simulink model "throttleMask"  (R2022b)
settings: Solver=ode45  StartTime=0.0  StopTime=20  RelTol=1e-3  EnableMultiTasking=on
PreLoadFcn:
  | % Throttle body parameters
  | etc_plant_data;
  | 
  | % Input data
  | load throttle_input;
settings Model: Creator=jrivitus  LastModifiedBy=bensweet
settings SolverCC: AlgebraicLoopSolver=TrustRegion
settings DataIOCC: ExternalInput=[t, duty, direction]  LimitDataPoints=on  LoadExternalInput=on  SaveFormat=Array  ReturnWorkspaceOutputs=off
settings OptimizationCC: ExpressionDepthLimit=2147483647  LifeSpan=inf
settings DebuggingCC: UnconnectedInputMsg=warning  UnconnectedOutputMsg=warning  UnconnectedLineMsg=warning  PregeneratedLibrarySubsystemCodeDiagnostic=none  SFMachineParentedDataDiag=warning
settings HardwareCC: ProdBitPerPointer=32  ProdBitPerSizeT=32  ProdBitPerPtrDiffT=32  ProdLargestAtomicFloat=None  ProdIntDivRoundTo=Undefined  ProdEndianess=Unspecified  ProdWordSize=32  ProdHWDeviceType=32-bit Generic
settings ModelReferenceCC: EnableRefExpFcnMdlSchedulingChecks=on  PropagateSignalLabelsOutOfModel=off
settings SFSimCC: SimUseLocalCustomCode=off
settings RTWCC: RTWUseLocalCustomCode=off  DLArmComputeVersion=19.05
settings CodeAppCC: StateflowObjectComments=on
settings GRTTargetCC: TargetLangStandard=C89/C90 (ANSI)  CombineOutputUpdateFcns=off  GRTInterface=on
settings ConfigComp: CovMetricSettings=dw  CovSaveCumulativeToWorkspaceVar=on  CovSaveSingleToWorkspaceVar=on  CovExternalEMLEnable=off  CovSFcnEnable=off

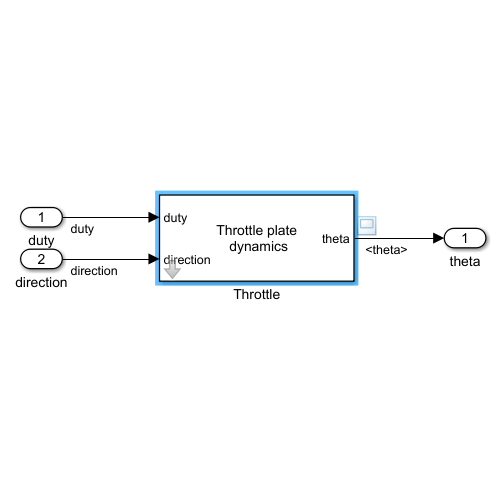
[thumbnail: Simulink's stored preview of the top-level diagram]
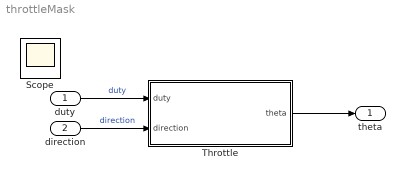
== system throttleMask ==
  duty : Inport
  direction : Inport  Port=2
  Throttle : Subsystem  mask(Throttle plate dynamics){J=2.45e-4, Km=3, Kd=0.03, Ks=0.2, theta_eq=pi/6}
      mask prompts: J "Inertia (J):"; Km "Motor torque constant (Km):"; Kd "Damping constant (Kd):"; Ks "Spring constant (Ks):"; theta_eq "Equilibrium angle (theta_eq):"
      mask help: Implements the dynamics for the throttle plate.
      mask Display: fprintf("Throttle plate\n dynamics")
  theta : Outport  VectorParamsAs1DForOutWhenUnconnected=off
  Scope : Scope
  wires:
  duty/1 -> Throttle/1(duty)  "duty"
  direction/1 -> Throttle/2(direction)  "direction"
  Throttle/1(theta) -> theta/1

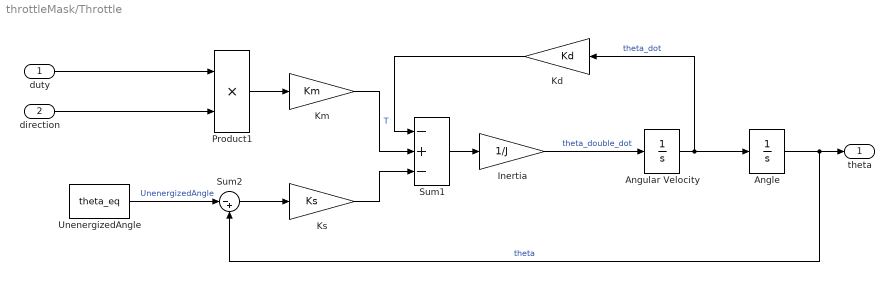
== system throttleMask/Throttle ==
  duty : Inport
  direction : Inport  Port=2
  Angle : Integrator  InitialCondition=pi/6  LimitOutput=on  UpperSaturationLimit=pi/2  LowerSaturationLimit=0
      settings: AttributesFormatString=Initial condition: %<InitialCondition>\n%<LowerSaturationLimit> <= theta <= %<UpperSaturationLimit>
  Angular Velocity : Integrator
      settings: AttributesFormatString=Initial condition: %<InitialCondition>
  Inertia : Gain  Gain=1/J  SaturateOnIntegerOverflow=on  OutDataTypeStr=Inherit: Same as input  ParamDataTypeStr=Inherit: Same as input
  Kd : Gain  Gain=Kd  SaturateOnIntegerOverflow=on  OutDataTypeStr=Inherit: Same as input  ParamDataTypeStr=Inherit: Same as input
  Km : Gain  Gain=Km  SaturateOnIntegerOverflow=on  OutDataTypeStr=Inherit: Same as input  ParamDataTypeStr=Inherit: Same as input
  Ks : Gain  Gain=Ks  SaturateOnIntegerOverflow=on  OutDataTypeStr=Inherit: Same as input  ParamDataTypeStr=Inherit: Same as input
  Product1 : Product  SaturateOnIntegerOverflow=on  OutDataTypeStr=Inherit: Same as first input
  Sum1 : Sum  Inputs=-+-  SaturateOnIntegerOverflow=on
  Sum2 : Sum  Inputs=|-+  SaturateOnIntegerOverflow=on
  UnenergizedAngle : Constant  Value=theta_eq
  theta : Outport  VectorParamsAs1DForOutWhenUnconnected=off
  wires:
  Product1/1 -> Km/1
  UnenergizedAngle/1 -> Sum2/1  "UnenergizedAngle"
  Sum2/1 -> Ks/1
  Angle/1 -> theta/1, Sum2/2  "theta"
  Angular Velocity/1 -> Angle/1, Kd/1  "theta_dot"
  Inertia/1 -> Angular Velocity/1  "theta_double_dot"
  Sum1/1 -> Inertia/1
  direction/1 -> Product1/2
  duty/1 -> Product1/1
  Km/1 -> Sum1/2  "T"
  Kd/1 -> Sum1/1
  Ks/1 -> Sum1/3
